simulink model "Modelling_Non_Linear_Equations"  (R2022b)
settings: Solver=VariableStepAuto  StartTime=0.0  StopTime=10.0  RelTol=1e-3
settings Model: Creator=tedro  LastModifiedBy=tedro

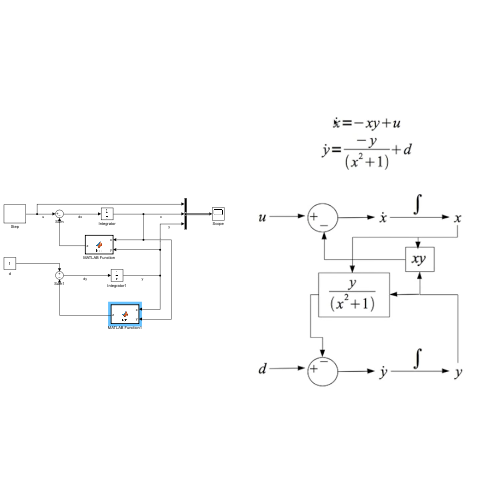
[thumbnail: Simulink's stored preview of the top-level diagram]
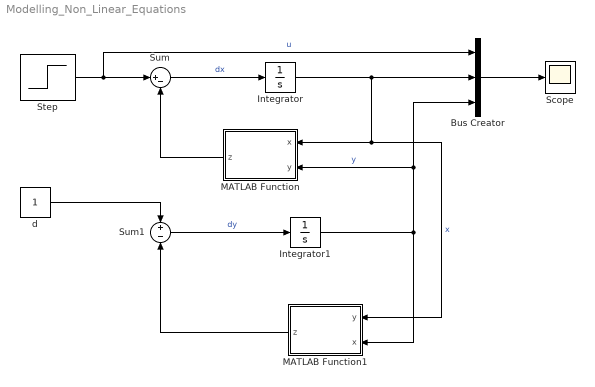
== system Modelling_Non_Linear_Equations ==
  Bus Creator : BusCreator  Inputs=3
  Integrator : Integrator
  Integrator1 : Integrator
  MATLAB Function : MATLAB Function  TreatAsAtomicUnit=on
  MATLAB Function1 : MATLAB Function  TreatAsAtomicUnit=on
  Scope : Scope
  Step : Step  SampleTime=0
  Sum : Sum  Inputs=|+-
  Sum1 : Sum  Inputs=+-
  d : Constant
  wires:
  Step/1 -> Bus Creator/1, Sum/1  "u"
  Sum/1 -> Integrator/1  "dx"
  Integrator/1 -> MATLAB Function1/1(y), MATLAB Function/1(x), Bus Creator/2  "x"
  d/1 -> Sum1/1
  Sum1/1 -> Integrator1/1  "dy"
  Integrator1/1 -> MATLAB Function1/2(x), MATLAB Function/2(y), Bus Creator/3  "y"
  MATLAB Function/1(z) -> Sum/2
  Bus Creator/1 -> Scope/1
  MATLAB Function1/1(z) -> Sum1/2

== matlab function Modelling_Non_Linear_Equations/MATLAB Function ==
  data: x input; z output; y input
function z = fcn(x,y)
z = x*y;

== matlab function Modelling_Non_Linear_Equations/MATLAB Function1 ==
  data: y input; x input; z output
function z = fcn(y,x)
z = y/(x^2 +1)
